simulink model "TST_BusCreatorForwardOptimization"  (Simulink 10.0)
settings: Solver=FixedStepDiscrete  StartTime=0.0  StopTime=10.0  FixedStep=0.02  RelTol=1e-3  EnableMultiTasking=on
settings Model: Creator=kharthforeign  LastModifiedBy=unknown
settings DataIOCC: LimitDataPoints=on  SignalLoggingSaveFormat=ModelDataLogs  SaveOutput=off  SignalLogging=off  SaveTime=off
settings OptimizationCC: BlockReduction=off  ConditionallyExecuteInputs=off  OptimizeBlockIOStorage=off  BufferReuse=off  GlobalBufferReuse=off  ExpressionFolding=off  ExpressionDepthLimit=2147483647  LocalBlockOutputs=off  InitFltsAndDblsToZero=on  OptimizeDataStoreBuffers=off  BusAssignmentInplaceUpdate=off
settings DebuggingCC: SolverPrmCheckMsg=warning  FcnCallInpInsideContextMsg=warning  StateNameClashWarn=warning
settings SFSimCC: SimParseCustomCode=off
settings GRTTargetCC: GeneratePreprocessorConditionals=Disable all
settings ConfigComp: CovExternalEMLEnable=off

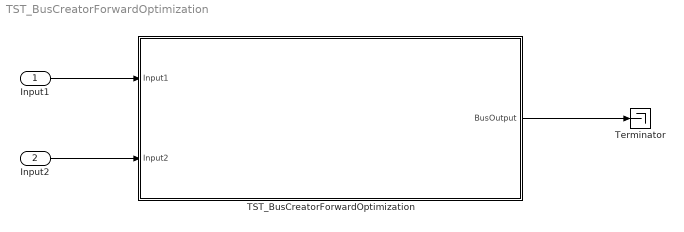
== system TST_BusCreatorForwardOptimization ==
  Input1 : Inport  OutDataTypeStr=double  BusOutputAsStruct=on
  Input2 : Inport  Port=2  OutDataTypeStr=uint32  PortDimensions=1  BusOutputAsStruct=on
  TST_BusCreatorForwardOptimization : Subsystem  TreatAsAtomicUnit=on
  Terminator : Terminator
  wires:
  Input1/1 -> TST_BusCreatorForwardOptimization/1(Input1)
  Input2/1 -> TST_BusCreatorForwardOptimization/2(Input2)
  TST_BusCreatorForwardOptimization/1(BusOutput) -> Terminator/1

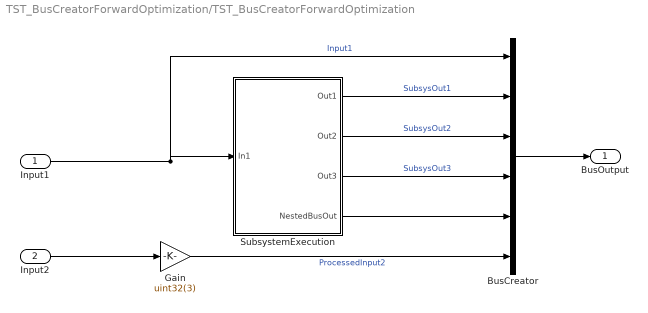
== system TST_BusCreatorForwardOptimization/TST_BusCreatorForwardOptimization ==
  Input1 : Inport  OutDataTypeStr=double  PortDimensions=1  BusOutputAsStruct=on
  Input2 : Inport  Port=2  OutDataTypeStr=uint32  PortDimensions=1  BusOutputAsStruct=on
  BusCreator : BusCreator  Inputs=6  NonVirtualBus=on
  Gain : Gain  Gain=uint32(3)  ParamDataTypeStr=uint32  OutDataTypeStr=uint32
  SubsystemExecution : Subsystem  TreatAsAtomicUnit=on
  BusOutput : Outport  BusOutputAsStruct=on
  wires:
  BusCreator/1 -> BusOutput/1
  Input1/1 -> SubsystemExecution/1(In1), BusCreator/1  "Input1"
  Input2/1 -> Gain/1
  SubsystemExecution/1(Out1) -> BusCreator/2  "SubsysOut1"
  SubsystemExecution/2(Out2) -> BusCreator/3  "SubsysOut2"
  SubsystemExecution/3(Out3) -> BusCreator/4  "SubsysOut3"
  Gain/1 -> BusCreator/6  "ProcessedInput2"
  SubsystemExecution/4(NestedBusOut) -> BusCreator/5

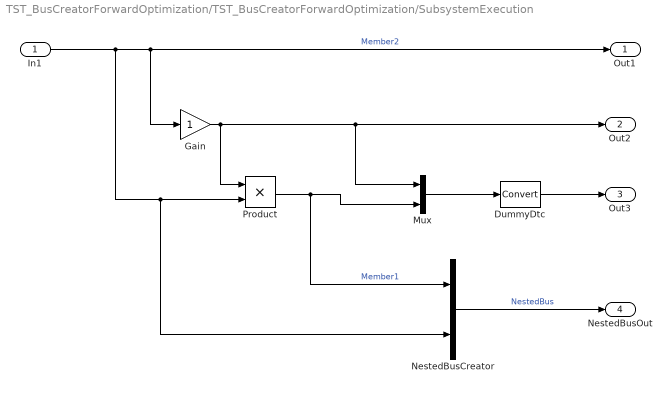
== system TST_BusCreatorForwardOptimization/TST_BusCreatorForwardOptimization/SubsystemExecution ==
  In1 : Inport
  DummyDtc : DataTypeConversion
  Gain : Gain
  Mux : Mux  Inputs=2
  NestedBusCreator : BusCreator  Inputs=2  NonVirtualBus=on
  Product : Product  RndMeth=Zero
  Out1 : Outport
  Out2 : Outport  Port=2
  Out3 : Outport  Port=3
  NestedBusOut : Outport  Port=4  BusOutputAsStruct=on
  wires:
  In1/1 -> Out1/1, Gain/1, Product/2, NestedBusCreator/2  "Member2"
  Gain/1 -> Product/1, Out2/1, Mux/1
  Mux/1 -> DummyDtc/1
  Product/1 -> Mux/2, NestedBusCreator/1  "Member1"
  DummyDtc/1 -> Out3/1
  NestedBusCreator/1 -> NestedBusOut/1  "NestedBus"
